simulink model "DoubleCap"  (R2022b)
settings: Solver=VariableStepAuto  StartTime=0.0  StopTime=3600  RelTol=1e-3
model workspace (MAT data in the model file):
  D = 45
  Tp = 0.001
undefined symbols (not defined in the file): Ion, Lithium
libraries: spsIdealSwitchLib x2, simulink x2, spsBatteryLib x1, spsParallelRLCBranchLib x1, spspowerguiLib x1
settings Model: Creator=MAAM  LastModifiedBy=MAAM
settings SolverCC: ZeroCrossAlgorithm=Adaptive
settings DebuggingCC: IgnoredZcDiagnostic=none

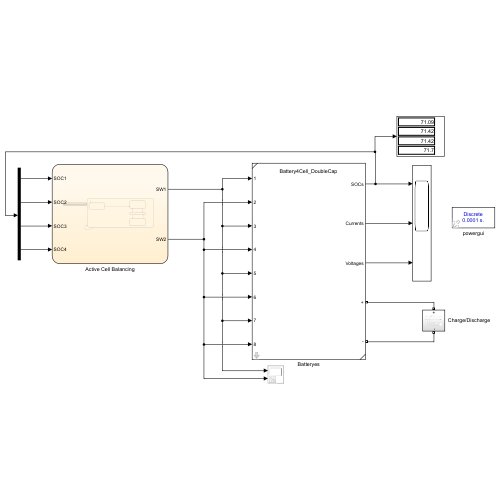
[thumbnail: Simulink's stored preview of the top-level diagram]
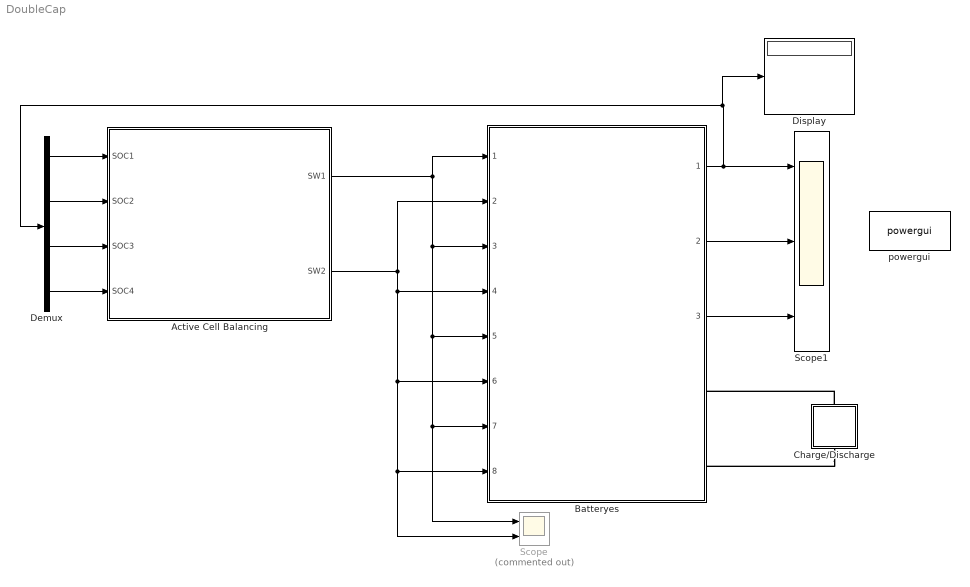
== system DoubleCap ==
  Active Cell Balancing : Stateflow chart  TreatAsAtomicUnit=on
  Batteryes : Subsystem  ReferencedSubsystem=Battery4Cell_DoubleCap  V0=3.7  Ah=2.6  SOC1=91  SOC2=96  SOC3=90  SOC4=98  C=50e-3
  Charge/Discharge : Subsystem
  Demux : Demux
  Display : Display
  Scope : Scope  Commented=on  NumInputPorts=2
  Scope1 : Scope  NumInputPorts=3
  powergui : spspowerguiLib/powergui  Priority=1  SimulationMode=Discrete  SampleTime=0.0001  frequency=60  Iterations=50  frequencyindice=0  Pbase=100e6  ErrMax=1e-4  UnitsV=kV  UnitsW=MW  buscounter=0  FunctionMessages=off  echomessages=off  EnableUseOfTLC=off  CurrentSourceSwitches=off  DisableSnubberDevices=off  DisableRonSwitches=off  DisableVfSwitches=off  DisplayEquations=off  AutomaticDiscreteSolvers=off  SolverType=Tustin/Backward Euler (TBE)  Interpol=off  ExternalGateDelay=off  methode=off  Ts=100  x0status=blocks  SPID=on  SwTol=0  HookPort=off  NonlinearTolerance=1e-4  nMaxIteration=100  ContinueOnMaxIteration=off  RestoreLinks=warning  ResistiveCurrentMeasurement=off  Frange=[0:2:500]  Ylog=off  Xlog=on  ShowGrid=off  save=off  variable=ZData  structure=0  ZoomFFT=off  StartTime=0.0  cycles=1  DisplayStyle=1  fundamental=60  FreqAxis=off  MaxFrequency=1000  frequencyindicesteady=1  RmsSteady=1  display=off
  wires:
  Batteryes/2 -> Scope1/2
  Batteryes/3 -> Scope1/3
  Batteryes/1 -> Demux/1, Display/1, Scope1/1
  Active Cell Balancing/1(SW1) -> Batteryes/7, Scope/1, Batteryes/5, Batteryes/3, Batteryes/1
  Active Cell Balancing/2(SW2) -> Batteryes/8, Scope/2, Batteryes/6, Batteryes/4, Batteryes/2
  Demux/1 -> Active Cell Balancing/1(SOC1)
  Demux/4 -> Active Cell Balancing/4(SOC4)
  Demux/3 -> Active Cell Balancing/3(SOC3)
  Demux/2 -> Active Cell Balancing/2(SOC2)
  connections:
  Charge/Discharge/RConn1 -- Batteryes/RConn2
  Charge/Discharge/LConn1 -- Batteryes/RConn1

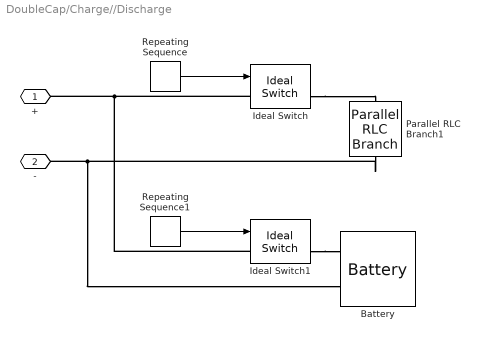
== system DoubleCap/Charge//Discharge ==
  Battery : spsBatteryLib/Battery  BatType=Lithium-Ion  ShowTempParam=off  ThermalPreset=no  ShowAgeParam=off  NomV=15  NomQ=100  SOC=100  Batt_Tr=30  PresetModel=on  MaxQ=100  MinV=11.25  FullV=17.4598  Dis_rate=43.4783  R=0.0015  Normal_OP=90.4348  expZone="[16.2058      4.91304]"  current=[6.5 13 32.5]  Units=Time  Tci=20  NomT=20  T2=-30  MaxQ2=4.8  FullV2=7.1  Normal_OP2=5.655  expZone2="[6.58           1]"  Rca=0.6  ti=2000  Dp=0  Neq0=0  Tsim=1e6  Ta1=25  Qeol=5.4*0.9  Reol=0.013333*1.2  Char_age=[2.3478, 3]  Dis_age=[2.3478, 10]  N1=1500  N2=10500  N3=1000  N4=1400  Ta2=45  N5=950
  Ideal Switch : spsIdealSwitchLib/Ideal Switch  Ron=0.0001  Lon=0  IC=0  Rs=1e7  Cs=inf  Measurements=on
  Ideal Switch1 : spsIdealSwitchLib/Ideal Switch  Ron=0.0001  Lon=0  IC=0  Rs=1e7  Cs=inf  Measurements=on
  Parallel RLC Branch1 : spsParallelRLCBranchLib/Parallel RLC Branch  LConnTagsString=a  RConnTagsString=__new0  BranchType=R  Resistance=1  Inductance=1e-3  SetiL0=off  InitialCurrent=0  Capacitance=1e-6  Setx0=off  InitialVoltage=0  Measurements=None
  Repeating Sequence : simulink/Sources/Repeating Sequence  rep_seq_t=[0 2400 2400.001 28000 28000.001]  rep_seq_y=[0 0 1 1 0]
  Repeating Sequence1 : simulink/Sources/Repeating Sequence  rep_seq_t=[0 2800 2800.001 3600 3600.001]  rep_seq_y=[0 0 1 1 0]
  + : PMIOPort  Side=Left
  - : PMIOPort  Port=2  Side=Right
  wires:
  Repeating Sequence1/1 -> Ideal Switch1/1
  Repeating Sequence/1 -> Ideal Switch/1
  connections:
  Ideal Switch1/RConn1 -- Battery/LConn1
  +/RConn1 -- Ideal Switch1/LConn1 -- Ideal Switch/LConn1
  -/RConn1 -- Battery/LConn2 -- Parallel RLC Branch1/RConn1
  Ideal Switch/RConn1 -- Parallel RLC Branch1/LConn1

== stateflow chart DoubleCap/Active Cell Balancing ==
  state Super
    state SW1_On
      en:
      SW1 = true;
      ex:
      SW1 = false;
      step = 1;
    state SW_Off
      en:
      SW1 = false;
      SW2 = false;
      step = 1;
    state SW_Wait
    state SW2_On
      en:
      SW2 = true;
      ex:
      SW2 = false;
      step = 2;
    (default) -> SW_Off
    SW_Off -> SW1_On : [getLowSOC(SOC1, SOC2, SOC3, SOC4) == true]
    SW_Wait -> SW1_On [order 1] : after((0.5-Don)/Freq, sec)[step >= 2]
    SW1_On -> SW_Wait : after(Don/Freq - 0.0001, sec)
    SW_Wait -> SW2_On [order 2] : after((0.5-Don)/Freq, sec)[step <= 1]
    SW2_On -> SW_Wait : after(Don/Freq - 0.0001, sec)
  state out  = getLowSOC(In1, In2, In3, In4) [function]
    (default) -> (junction 2) : {out = max(In1, In2, In3, In4)  - min(In1, In2, In3, In4); }
    (junction 2) -> (junction 21) [order 1] : [out > threshold]
    (junction 2) -> (junction 26) [order 2] : {out = false;}
    (junction 21) -> (junction 24) : {out = true;}
    (junction 24) -> (junction 26)
    (junction 26) -> (junction 130)
  Super -> Super : [getLowSOC(SOC1, SOC2, SOC3, SOC4) == false]
  data: In1 function_input double size=1; In2 function_input double size=1; In3 function_input double size=1; In4 function_input double size=1; out function_output double size=1; SOC1 input double size=1; SOC2 input double size=1; SOC3 input double size=1; SOC4 input double size=1; SW1 output size=1; SW2 output size=1; Don constant double =0.45; Freq constant double =1000; threshold constant double =0.5; step local double
